simulink model "full_maneuver_platoon"  (R2022a)
settings: Solver=ode23t  StartTime=0.0  StopTime=300  FixedStep=0.1  MaxStep=0.01  RelTol=1e-3
InitFcn:
  | totalVehicles = 7;
  | if exist('vehStatesBus', 'var')==0
  | load vehBuses
  | end
  | if exist('vehErrorsBus', 'var')==0
  | load vehBuses
  | end
libraries: simulink x80, powerlib_meascontrol x16, autolibshared x7, dspsigops x4
(part 5 of 9)

== system full_maneuver_platoon/p2/CACC destination lane/Virtual Vehicle Following ==
  ego : Inport
  virtualLeader : Inport  Port=2
  leaderChange : Inport  Port=3
  extraSpaceFlag : Inport  Port=4
  Bus Selector : BusSelector  OutputSignals=u
  Compute Errors : Subsystem
  Define Desired Distance : Subsystem
  Min Velocity Control : Subsystem  TreatAsAtomicUnit=on
  NOT : Logic  Operator=NOT  IconShape=distinctive  AllPortsSameDT=off  OutDataTypeStr=boolean
  Scope : Scope  NumInputPorts=2
  Switch : Switch  Criteria=u2 > Threshold  SaturateOnIntegerOverflow=off  InputSameDT=off
  Terminator : Terminator
  Velocity Error : Subsystem
  Virtual Leader Following : Subsystem  TreatAsAtomicUnit=on
  comf saturation : Saturate  UpperLimit=maxComfAccel  LowerLimit=minComfAccel
  comf jerk : RateLimiter  RisingSlewLimit=maxComfJerk  FallingSlewLimit=minComfJerk  SampleTimeMode=inherited
  switch min vel : Subsystem
  vMin : Constant  Value=vMin
  u : Outport  InitialOutput=0  VectorParamsAs1DForOutWhenUnconnected=off
  virtualErrors : Outport  Port=2  OutputWhenDisabled=reset  InitialOutput=[0, 0]  VectorParamsAs1DForOutWhenUnconnected=off
  virtualGap : Outport  Port=3  OutputWhenDisabled=reset  InitialOutput=[0]  VectorParamsAs1DForOutWhenUnconnected=off
  wires:
  Switch/1 -> Scope/2, comf saturation/1
  comf jerk/1 -> u/1
  comf saturation/1 -> comf jerk/1
  Bus Selector/1 -> Virtual Leader Following/3(realInput)  "<u>"
  Velocity Error/2(ea) -> Min Velocity Control/2(ea)
  Velocity Error/1(ev) -> Min Velocity Control/1(ev)
  NOT/1 -> Switch/2, Scope/1, Virtual Leader Following/5(inRange)
  switch min vel/1(inRange) -> NOT/1, Min Velocity Control/3(intergralReset), Velocity Error/3(filterReset)
  extraSpaceFlag/1 -> Define Desired Distance/1(extraSpaceFlag)
  Min Velocity Control/1(u) -> Switch/3  "uMinVelControl"
  Compute Errors/3("gap ") -> virtualGap/1, switch min vel/3(gap)
  Virtual Leader Following/1(u) -> Switch/1  "uVehFoll"
  ego/1 -> Compute Errors/1(ego), Bus Selector/1, Velocity Error/1(ego)
  vMin/1 -> switch min vel/6(vRef), Velocity Error/2(velRef)
  Compute Errors/1(errors) -> switch min vel/1(errors), Virtual Leader Following/1(errors), virtualErrors/1
  virtualLeader/1 -> Compute Errors/2(leader)
  leaderChange/1 -> Compute Errors/5(velFilterReset), Virtual Leader Following/4(leaderChange)
  Compute Errors/4(unsafeFlag) -> Terminator/1
  Compute Errors/2(errorsDot) -> Virtual Leader Following/2(errorsDot), switch min vel/2(errorsDot)
  Define Desired Distance/1(h) -> switch min vel/4(h), Compute Errors/3(h)
  Define Desired Distance/2(d0) -> switch min vel/5(d0), Compute Errors/4(d0)

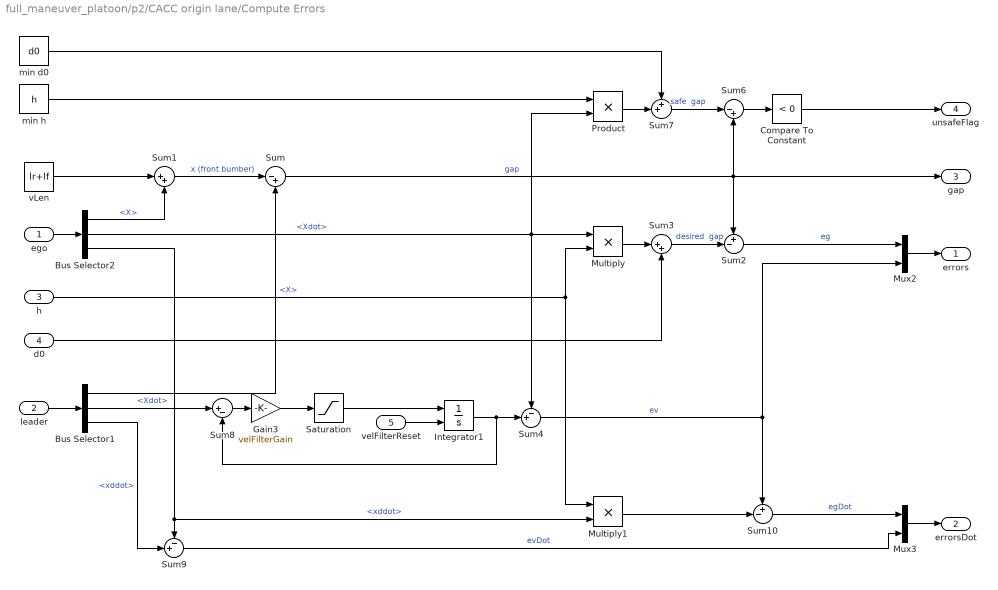
== system full_maneuver_platoon/p2/CACC origin lane/Compute Errors ==
  ego : Inport
  leader : Inport  Port=2
  h : Inport  Port=3
  d0 : Inport  Port=4
  velFilterReset : Inport  Port=5
  Bus Selector1 : BusSelector  OutputSignals=X,Xdot,xddot
  Bus Selector2 : BusSelector  OutputSignals=X,Xdot,xddot
  Compare To Constant : simulink/Logic and Bit Operations/Compare To Constant  relop=<  const=0  OutDataTypeStr=boolean
  Gain3 : Gain  Gain=velFilterGain
  Integrator1 : Integrator  ExternalReset=rising  InitialCondition=vx0
  Multiply : Product
  Multiply1 : Product
  Mux2 : Mux  Inputs=2
  Mux3 : Mux  Inputs=2
  Product : Product
  Saturation : Saturate  UpperLimit=maxAcceleration  LowerLimit=minAcceleration
  Sum : Sum  Inputs=|-+
  Sum1 : Sum  Inputs=|++
  Sum10 : Sum  Inputs=+-|
  Sum2 : Sum  Inputs=+-|
  Sum3 : Sum  Inputs=|++
  Sum4 : Sum  Inputs=-+|
  Sum6 : Sum  Inputs=|-+
  Sum7 : Sum  Inputs=++|
  Sum8 : Sum  Inputs=|+-
  Sum9 : Sum  Inputs=-+|
  min d0 : Constant  Value=d0
  min h : Constant  Value=h
  vLen : Constant  Value=lr+lf
  errors : Outport  VectorParamsAs1DForOutWhenUnconnected=off
  errorsDot : Outport  Port=2
  "gap " : Outport  Port=3  VectorParamsAs1DForOutWhenUnconnected=off
  unsafeFlag : Outport  Port=4  VectorParamsAs1DForOutWhenUnconnected=off
  wires:
  Mux2/1 -> errors/1
  velFilterReset/1 -> Integrator1/2
  Sum6/1 -> Compare To Constant/1
  Sum7/1 -> Sum6/1  "safe  gap"
  min h/1 -> Product/1
  Compare To Constant/1 -> unsafeFlag/1
  Sum2/1 -> Mux2/1  "eg"
  Bus Selector1/1 -> Sum/2  "<X>"
  Product/1 -> Sum7/2
  Sum3/1 -> Sum2/2  "desired  gap"
  Sum1/1 -> Sum/1  "x (front bumber)"
  Bus Selector2/2 -> Sum4/1, Multiply/1, Product/2  "<Xdot>"
  d0/1 -> Sum3/2
  vLen/1 -> Sum1/1
  min d0/1 -> Sum7/1
  Multiply/1 -> Sum3/1
  Sum/1 -> Sum2/1, Sum6/2, "gap "/1  "gap"
  Bus Selector2/1 -> Sum1/2  "<X>"
  h/1 -> Multiply/2, Multiply1/1
  Bus Selector1/2 -> Sum8/1  "<Xdot>"
  Sum4/1 -> Mux2/2, Sum10/1  "ev"
  Gain3/1 -> Saturation/1
  Saturation/1 -> Integrator1/1
  Integrator1/1 -> Sum4/2, Sum8/2
  Sum8/1 -> Gain3/1
  Bus Selector1/3 -> Sum9/2  "<xddot>"
  Bus Selector2/3 -> Sum9/1, Multiply1/2  "<xddot>"
  Multiply1/1 -> Sum10/2
  Sum10/1 -> Mux3/1  "egDot"
  Sum9/1 -> Mux3/2  "evDot"
  Mux3/1 -> errorsDot/1
  ego/1 -> Bus Selector2/1
  leader/1 -> Bus Selector1/1

== system full_maneuver_platoon/p2/CACC origin lane/Define Desired Distance ==
  extraSpaceFlag : Inport
  Constant : Constant  Value=h
  Constant1 : Constant  Value=d0
  Constant2 : Constant  Value=hLC
  Constant3 : Constant  Value=d0LC
  Demux : Demux  Outputs=2
  Integrator : Integrator  InitialCondition=[h d0]
  Mux : Mux  Inputs=2
  Mux1 : Mux  Inputs=2
  Saturation1 : Saturate  UpperLimit=hFilterSaturation/2  LowerLimit=-hFilterSaturation
  Sum5 : Sum  Inputs=|+-
  Switch : Switch  Criteria=u2 > Threshold  SaturateOnIntegerOverflow=off  InputSameDT=off
  hFilterGain : Gain  Gain=hFilterGain
  h : Outport
  d0 : Outport  Port=2
  wires:
  Mux/1 -> Switch/3
  Constant/1 -> Mux/1
  hFilterGain/1 -> Saturation1/1
  Constant2/1 -> Mux1/1
  Sum5/1 -> hFilterGain/1
  Mux1/1 -> Switch/1
  Switch/1 -> Sum5/1
  Constant3/1 -> Mux1/2
  Constant1/1 -> Mux/2
  extraSpaceFlag/1 -> Switch/2
  Saturation1/1 -> Integrator/1
  Integrator/1 -> Demux/1, Sum5/2
  Demux/1 -> h/1
  Demux/2 -> d0/1

== system full_maneuver_platoon/p2/CACC origin lane/Veh Following ==
  errors : Inport
  errorsDot : Inport  Port=2
  realInput : Inport  Port=3
  leaderChange : Inport  Port=4
  inRange : Inport  Port=5
  AND : Logic  IconShape=distinctive  AllPortsSameDT=off  OutDataTypeStr=boolean
  Compare To Constant : simulink/Logic and Bit Operations/Compare To Constant  relop=~=  const=0  OutDataTypeStr=boolean
  Constant : Constant  Value=Ki
  Demux : Demux  Outputs=2
  Demux1 : Demux  Outputs=2
  Gain : Gain  Gain=Ka
  Gain1 : Gain  Gain=Kdd
  Gain3 : Gain  Commented=on  Gain=10
  Integrator1 : Integrator  Commented=on  ExternalReset=either  InitialConditionSource=external  InitialCondition=vx0
  Kd : Gain  Gain=Kd
  Kp : Gain  Gain=Kp
  Saturation : Saturate  Commented=on  UpperLimit=maxComfAccel  LowerLimit=minAcceleration
  Saturation1 : Saturate  UpperLimit=maxGapError  LowerLimit=minGapError
  Scope : Scope  NumInputPorts=6
  Sum : Sum  Inputs=+-|
  Sum1 : Sum  Inputs=+++++
  Sum8 : Sum  Commented=on  Inputs=|+-
  Transport Delay : TransportDelay  DelayTime=0.1
  integralTerm : Subsystem
  u : Outport  VectorParamsAs1DForOutWhenUnconnected=off
  wires:
  AND/1 -> integralTerm/Enable
  inRange/1 -> Integrator1/2, AND/2
  Compare To Constant/1 -> AND/1
  Constant/1 -> Compare To Constant/1
  Kp/1 -> Sum1/2, Scope/2
  Gain3/1 -> Saturation/1
  Sum8/1 -> Gain3/1
  Saturation/1 -> Integrator1/1
  Integrator1/1 -> Sum8/2
  errors/1 -> Demux/1
  Saturation1/1 -> integralTerm/1(eh), Kp/1
  Demux/2 -> Kd/1  "ev"
  Kd/1 -> Sum1/3, Scope/3
  Demux/1 -> Saturation1/1  "eg"
  leaderChange/1 -> integralTerm/3(leaderChange)
  Transport Delay/1 -> Sum1/1, Scope/1
  realInput/1 -> Sum/2, Integrator1/3
  Sum/1 -> integralTerm/2(inputDiff)
  integralTerm/1(Out1) -> Transport Delay/1
  Gain1/1 -> Sum1/4, Scope/4
  Gain/1 -> Sum1/5, Scope/5
  Sum1/1 -> Sum8/1, Sum/1, Scope/6, u/1
  errorsDot/1 -> Demux1/1
  Demux1/1 -> Gain1/1  "egDot"
  Demux1/2 -> Gain/1  "evDot"

== system full_maneuver_platoon/p2/CACC origin lane/Velocity Control ==
  ev : Inport
  ea : Inport  Port=2
  integralReset : Inport  Port=3
  Abs : Abs  SaturateOnIntegerOverflow=off
  Compare To Constant : simulink/Logic and Bit Operations/Compare To Constant  relop=<  const=maxComfAccel*2  OutDataTypeStr=boolean
  Gain : Gain  Gain=velKd
  Scope : Scope  NumInputPorts=4
  Scope1 : Scope  NumInputPorts=2
  Sum3 : Sum  Inputs=+++
  Transport Delay : TransportDelay  DelayTime=0.1
  integral term : Subsystem
  velKp : Gain  Gain=velKp
  u : Outport  VectorParamsAs1DForOutWhenUnconnected=off
  wires:
  integralReset/1 -> integral term/2(integralReset)
  Sum3/1 -> Transport Delay/1, Scope/4, u/1
  Gain/1 -> Sum3/3, Scope/3  "derivative"
  ea/1 -> Gain/1
  velKp/1 -> Sum3/2, Scope/2  "proportional"
  ev/1 -> integral term/1(ev), velKp/1
  Abs/1 -> Compare To Constant/1
  integral term/1(Out1) -> Scope/1, Sum3/1  "integral"
  Compare To Constant/1 -> Scope1/2, integral term/Enable
  Transport Delay/1 -> Abs/1, Scope1/1

== system full_maneuver_platoon/p2/CACC origin lane/Velocity Error ==
  ego : Inport
  velRef : Inport  Port=2
  filterReset : Inport  Port=3
  Bus Selector : BusSelector  OutputSignals=Xdot,xddot
  Gain1 : Gain  Gain=velFilterGain
  Gain3 : Gain  Gain=velFilterGain
  Integrator1 : Integrator  ExternalReset=rising  InitialConditionSource=external  InitialCondition=vx0
  Saturation : Saturate  UpperLimit=maxComfAccel  LowerLimit=minComfAccel
  Saturation1 : Saturate  UpperLimit=maxComfAccel  LowerLimit=minComfAccel
  Scope : Scope  NumInputPorts=2
  Scope1 : Scope  NumInputPorts=2
  Sum : Sum  Inputs=+-|
  Sum1 : Sum  Inputs=-+|
  Sum2 : Sum  Inputs=+-|
  Sum8 : Sum  Inputs=|+-
  ev : Outport
  ea : Outport  Port=2
  wires:
  Saturation1/1 -> Sum2/1
  Gain1/1 -> Saturation1/1
  Sum1/1 -> Gain1/1  "filter error"
  Bus Selector/2 -> Sum2/2  "<xddot>"
  Sum2/1 -> ea/1, Scope/2
  Sum8/1 -> Gain3/1
  Gain3/1 -> Saturation/1
  Saturation/1 -> Integrator1/1
  velRef/1 -> Sum8/1, Sum1/2, Scope1/1
  Integrator1/1 -> Sum/1, Sum8/2, Sum1/1, Scope1/2
  ego/1 -> Bus Selector/1
  Bus Selector/1 -> Integrator1/3, Sum/2  "<Xdot>"
  Sum/1 -> ev/1, Scope/1
  filterReset/1 -> Integrator1/2

== system full_maneuver_platoon/p2/CACC origin lane/switch free flow ==
  errors : Inport
  errorsDot : Inport  Port=2
  gap : Inport  Port=3
  h : Inport  Port=4
  d0 : Inport  Port=5
  vRef : Inport  Port=6
  Demux1 : Demux  Outputs=2
  Gain1 : Gain
  MATLAB Function : MATLAB Function  TreatAsAtomicUnit=on
  Relay : Relay  OnSwitchValue=1  OffSwitchValue=-1
  Scope : Scope  NumInputPorts=3
  Selector : Selector  InputPortWidth=2  IndexOptions=Index vector (dialog)  Indices=[2]  OutputSizes=1
  Sum2 : Sum  Inputs=-+
  inRange : Outport  VectorParamsAs1DForOutWhenUnconnected=off
  wires:
  d0/1 -> MATLAB Function/2(d0)
  vRef/1 -> MATLAB Function/3(vRef)
  h/1 -> Gain1/1
  errors/1 -> Selector/1
  gap/1 -> Scope/1, Sum2/1
  Sum2/1 -> Relay/1
  Selector/1 -> MATLAB Function/4(ev)
  Relay/1 -> inRange/1, Scope/3
  Gain1/1 -> MATLAB Function/1(h)
  MATLAB Function/1(maxGap) -> Sum2/2, Scope/2
  errorsDot/1 -> Demux1/1
  Demux1/1 -> MATLAB Function/5(ehDot)
  Demux1/2 -> MATLAB Function/6(ea)

== system full_maneuver_platoon/p2/Find Leader/Subsystem ==
  ego : Inport
  all : Inport  Port=2
  Enable : EnablePort
  MATLAB Function : MATLAB Function  TreatAsAtomicUnit=on
  idx : Outport  InitialOutput=1  VectorParamsAs1DForOutWhenUnconnected=off
  wires:
  all/1 -> MATLAB Function/2(allVehicles)
  MATLAB Function/1(leaderIdx) -> idx/1
  ego/1 -> MATLAB Function/1(ego)

== system full_maneuver_platoon/p2/Find Leader/farAwayVeh ==
  ego : Inport  OutDataTypeStr=Bus: vehStatesBus
  Bus Assignment : BusAssignment  AssignedSignals=X
  Bus Selector : BusSelector  OutputSignals=X
  Constant : Constant  Value=1000
  Sum : Sum  Inputs=|++
  Out1 : Outport  OutDataTypeStr=Bus: vehStatesBus  VectorParamsAs1DForOutWhenUnconnected=off
  wires:
  Sum/1 -> Bus Assignment/2  "X"
  Bus Selector/1 -> Sum/1  "<X>"
  Bus Assignment/1 -> Out1/1
  Constant/1 -> Sum/2
  ego/1 -> Bus Selector/1, Bus Assignment/1

== system full_maneuver_platoon/p2/Lane Change Strategy/Strategy 1: synchronous ==
  gapRequest : Inport
  lcFlag : Inport  Port=2
  positionInPlatoon : Inport  Port=3
  platoonStates : Inport  Port=4
  isLaneChangeSafe : Inport  Port=5
  isLaneChangeDone : Inport  Port=6
  isGapClosed : Inport  Port=7
  realCACCstate : Inport  Port=8
  Chart : Stateflow chart  TreatAsAtomicUnit=on
      settings: PortSchema="{\"entries\":[{\"content\":{\"sides\":[{\"content\":{\"connectorIds\":[\"In1\",\"In2\",\"In3\",\"In4\",\"In6\",\"In5\",\"In7\",\"In8\"]},\"type\":\"ConnectorPlacement.EquallySpacedRectSide\",\"uuid\":\"395656aa-3e0f-49ff-a8a2-bf7c57c42e6d\"},{\"content\":{\"connectorIds\":[\"Out1\",\"Out2\",\"Out3\",\"Out4\",\"Out5\"],\"side\":\"RIGHT\"},\"type\":\"ConnectorPlacement.EquallySpacedRectSide\",\"uuid\":\"d914af52-9e9a-4b17-a1e4-773e769de9a6\"},{\"content\":{\"connectorIds\":[],\"side\":\"TOP\"},\"type\":\"ConnectorPlacement.EquallySpacedRectSide\",\"uuid\":\"e4221941-8de7-47a5-9bcd-f17ee6e4f42c\"}]},\"type\":\"ConnectorPlacement.EquallySpacedConnector\",\"uuid\":\"61bad5e0-e673-4247-b49d-1296c33c05b0\"}],\"packageUris\":[\"http://schema.mathworks.com/mf0/Connector/19700101\"],\"version\":\"1.0\"}"
  Sum : Sum  Inputs=|++
  Width : Width
  determine virtual follower idx : Subsystem  TreatAsAtomicUnit=on
  determine virtual leader idx : Subsystem
  number of non-lane changing vehicles : Constant  Value=4
  maneuverState : Outport
  mustIncreaseGap : Outport  Port=2
  canStartLaneChange : Outport  Port=3
  hasVirtualLeader : Outport  Port=4
  virtualLeaderIdx : Outport  Port=5
  virtualFollowerIdx : Outport  Port=6
  wires:
  Sum/1 -> determine virtual leader idx/1(nVehicles)
  Width/1 -> Sum/1
  number of non-lane changing vehicles/1 -> Sum/2
  determine virtual leader idx/1(virtualLeaderIdx) -> virtualLeaderIdx/1
  determine virtual follower idx/1(virtualFollowerIdx) -> virtualFollowerIdx/1
  isLaneChangeDone/1 -> Chart/5(isLaneChangeDone)
  positionInPlatoon/1 -> Chart/3(positionInPlatoon)
  isLaneChangeSafe/1 -> Chart/6(isLaneChangeSafe)
  lcFlag/1 -> Chart/2(hasLaneChangeIntention), determine virtual leader idx/2(lcFlag)
  Chart/2(mustIncreaseGap) -> mustIncreaseGap/1
  Chart/1(maneuverState) -> maneuverState/1
  platoonStates/1 -> Chart/4(platoonStates), Width/1
  isGapClosed/1 -> Chart/7(isGapClosed)
  Chart/3(canStartLaneChange) -> canStartLaneChange/1
  Chart/5(hasVirtualFollower) -> determine virtual follower idx/Enable
  Chart/4(hasVirtualLeader) -> determine virtual leader idx/Enable, hasVirtualLeader/1
  gapRequest/1 -> Chart/1(gapRequest)
  realCACCstate/1 -> Chart/8(realCACCstate)

== system full_maneuver_platoon/p2/Lane Change Strategy/Strategy 2: leader first ==
  gapRequest : Inport
  lcFlag : Inport  Port=2
  positionInPlatoon : Inport  Port=3
  platoonStates : Inport  Port=4
  isLaneChangeSafe : Inport  Port=5
  isLaneChangeDone : Inport  Port=6
  isGapClosed : Inport  Port=7
  realCACCstate : Inport  Port=8
  Chart : Stateflow chart  TreatAsAtomicUnit=on
      settings: PortSchema="{\"entries\":[{\"content\":{\"sides\":[{\"content\":{\"connectorIds\":[\"In1\",\"In2\",\"In3\",\"In5\",\"In4\",\"In6\",\"In7\",\"In8\"]},\"type\":\"ConnectorPlacement.EquallySpacedRectSide\",\"uuid\":\"395656aa-3e0f-49ff-a8a2-bf7c57c42e6d\"},{\"content\":{\"connectorIds\":[\"Out1\",\"Out2\",\"Out3\",\"Out4\",\"Out5\"],\"side\":\"RIGHT\"},\"type\":\"ConnectorPlacement.EquallySpacedRectSide\",\"uuid\":\"d914af52-9e9a-4b17-a1e4-773e769de9a6\"},{\"content\":{\"connectorIds\":[],\"side\":\"TOP\"},\"type\":\"ConnectorPlacement.EquallySpacedRectSide\",\"uuid\":\"e4221941-8de7-47a5-9bcd-f17ee6e4f42c\"}]},\"type\":\"ConnectorPlacement.EquallySpacedConnector\",\"uuid\":\"61bad5e0-e673-4247-b49d-1296c33c05b0\"}],\"packageUris\":[\"http://schema.mathworks.com/mf0/Connector/19700101\"],\"version\":\"1.0\"}"
  Sum : Sum  Inputs=|++
  Width : Width
  determine virtual follower idx : Subsystem  TreatAsAtomicUnit=on
  determine virtual leader idx : Subsystem
  number of non-lane changing vehicles : Constant  Value=4
  maneuverState : Outport
  mustIncreaseGap : Outport  Port=2
  canStartLaneChange : Outport  Port=3
  hasVirtualLeader : Outport  Port=4
  virtualLeaderIdx : Outport  Port=5
  virtualFollowerIdx : Outport  Port=6
  wires:
  number of non-lane changing vehicles/1 -> Sum/2
  Sum/1 -> determine virtual leader idx/1(nVehicles)
  Width/1 -> Sum/1
  determine virtual leader idx/1(virtualLeaderIdx) -> virtualLeaderIdx/1
  determine virtual follower idx/1(virtualFollowerIdx) -> virtualFollowerIdx/1
  isLaneChangeDone/1 -> Chart/5(isLaneChangeDone)
  positionInPlatoon/1 -> determine virtual leader idx/3(posInPlatoon), Chart/3(positionInPlatoon)
  isLaneChangeSafe/1 -> Chart/6(isLaneChangeSafe)
  lcFlag/1 -> determine virtual leader idx/2(lcFlag), Chart/2(hasLaneChangeIntention)
  Chart/2(mustIncreaseGap) -> mustIncreaseGap/1
  Chart/1(maneuverState) -> maneuverState/1
  platoonStates/1 -> Width/1, Chart/4(platoonStates)
  isGapClosed/1 -> Chart/7(isGapClosed)
  Chart/3(canStartLaneChange) -> canStartLaneChange/1
  Chart/5(hasVirtualFollower) -> determine virtual follower idx/Enable
  Chart/4(hasVirtualLeader) -> determine virtual leader idx/Enable, hasVirtualLeader/1
  gapRequest/1 -> Chart/1(gapRequest)
  realCACCstate/1 -> Chart/8(realCACCstate)

== system full_maneuver_platoon/p2/Lane Change Strategy/Strategy 3: last first ==
  gapRequest : Inport
  lcFlag : Inport  Port=2
  positionInPlatoon : Inport  Port=3
  platoonStates : Inport  Port=4
  isLaneChangeSafe : Inport  Port=5
  isLaneChangeDone : Inport  Port=6
  isGapClosed : Inport  Port=7
  realCACCstate : Inport  Port=8
  Chart : Stateflow chart  TreatAsAtomicUnit=on
      settings: PortSchema="{\"entries\":[{\"content\":{\"sides\":[{\"content\":{\"connectorIds\":[\"In1\",\"In2\",\"In3\",\"In4\",\"In6\",\"In5\",\"In7\",\"In8\"]},\"type\":\"ConnectorPlacement.EquallySpacedRectSide\",\"uuid\":\"395656aa-3e0f-49ff-a8a2-bf7c57c42e6d\"},{\"content\":{\"connectorIds\":[\"Out1\",\"Out2\",\"Out3\",\"Out4\",\"Out5\"],\"side\":\"RIGHT\"},\"type\":\"ConnectorPlacement.EquallySpacedRectSide\",\"uuid\":\"d914af52-9e9a-4b17-a1e4-773e769de9a6\"},{\"content\":{\"connectorIds\":[],\"side\":\"TOP\"},\"type\":\"ConnectorPlacement.EquallySpacedRectSide\",\"uuid\":\"e4221941-8de7-47a5-9bcd-f17ee6e4f42c\"}]},\"type\":\"ConnectorPlacement.EquallySpacedConnector\",\"uuid\":\"61bad5e0-e673-4247-b49d-1296c33c05b0\"}],\"packageUris\":[\"http://schema.mathworks.com/mf0/Connector/19700101\"],\"version\":\"1.0\"}"
  Sum : Sum
  Width : Width
  determine virtual follower idx : Subsystem
  determine virtual leader idx : Subsystem
  number of non-lane changing vehicles : Constant  Value=4
  maneuverState : Outport
  mustIncreaseGap : Outport  Port=2
  canStartLaneChange : Outport  Port=3
  hasVirtualLeader : Outport  Port=4
  virtualLeaderIdx : Outport  Port=5
  virtualFollowerIdx : Outport  Port=6
  wires:
  Sum/1 -> determine virtual leader idx/1(nVehicles)
  number of non-lane changing vehicles/1 -> Sum/2
  determine virtual leader idx/1(virtualLeaderIdx) -> virtualLeaderIdx/1
  determine virtual follower idx/1(virtual follower idx) -> virtualFollowerIdx/1
  Width/1 -> determine virtual follower idx/1(platoonSize), Sum/1
  isLaneChangeDone/1 -> determine virtual leader idx/3(lcDone), Chart/5(isLaneChangeDone)
  positionInPlatoon/1 -> determine virtual follower idx/2(posInPlatoon), determine virtual leader idx/4(posInPlatoon), Chart/3(positionInPlatoon)
  isLaneChangeSafe/1 -> Chart/6(isLaneChangeSafe)
  lcFlag/1 -> determine virtual leader idx/2(lcFlag), Chart/2(hasLaneChangeIntention)
  Chart/2(mustIncreaseGap) -> mustIncreaseGap/1
  Chart/1(maneuverState) -> maneuverState/1
  platoonStates/1 -> Width/1, Chart/4(platoonStates)
  isGapClosed/1 -> Chart/7(isGapClosed)
  Chart/3(canStartLaneChange) -> canStartLaneChange/1
  Chart/5(hasVirtualFollower) -> determine virtual follower idx/Enable
  Chart/4(hasVirtualLeader) -> determine virtual leader idx/Enable, hasVirtualLeader/1
  gapRequest/1 -> Chart/1(gapRequest)
  realCACCstate/1 -> Chart/8(realCACCstate)

== system full_maneuver_platoon/p2/Lane Change Strategy/Strategy 4: leader first invert ==
  gapRequest : Inport
  lcFlag : Inport  Port=2
  positionInPlatoon : Inport  Port=3
  platoonStates : Inport  Port=4
  isLaneChangeSafe : Inport  Port=5
  isLaneChangeDone : Inport  Port=6
  isGapClosed : Inport  Port=7
  realCACCstate : Inport  Port=8
  Chart : Stateflow chart  TreatAsAtomicUnit=on
      settings: PortSchema="{\"entries\":[{\"content\":{\"sides\":[{\"content\":{\"connectorIds\":[\"In1\",\"In2\",\"In3\",\"In4\",\"In6\",\"In5\",\"In7\",\"In8\"]},\"type\":\"ConnectorPlacement.EquallySpacedRectSide\",\"uuid\":\"395656aa-3e0f-49ff-a8a2-bf7c57c42e6d\"},{\"content\":{\"connectorIds\":[\"Out1\",\"Out2\",\"Out3\",\"Out4\",\"Out5\"],\"side\":\"RIGHT\"},\"type\":\"ConnectorPlacement.EquallySpacedRectSide\",\"uuid\":\"d914af52-9e9a-4b17-a1e4-773e769de9a6\"},{\"content\":{\"connectorIds\":[],\"side\":\"TOP\"},\"type\":\"ConnectorPlacement.EquallySpacedRectSide\",\"uuid\":\"e4221941-8de7-47a5-9bcd-f17ee6e4f42c\"}]},\"type\":\"ConnectorPlacement.EquallySpacedConnector\",\"uuid\":\"61bad5e0-e673-4247-b49d-1296c33c05b0\"}],\"packageUris\":[\"http://schema.mathworks.com/mf0/Connector/19700101\"],\"version\":\"1.0\"}"
  Subsystem : Subsystem
  Subsystem1 : Subsystem
  Sum : Sum  Inputs=++|
  Width : Width
  number of non-lane changing vehicles : Constant  Value=4
  maneuverState : Outport
  mustIncreaseGap : Outport  Port=2
  canStartLaneChange : Outport  Port=3
  hasVirtualLeader : Outport  Port=4
  virtualLeaderIdx : Outport  Port=5
  virtualFollowerIdx : Outport  Port=6
  wires:
  Subsystem1/1(virtualLeaderIdx) -> virtualLeaderIdx/1
  Sum/1 -> Subsystem1/1(nVehicles)
  Width/1 -> Sum/2
  number of non-lane changing vehicles/1 -> Sum/1
  Subsystem/1(virtualFollowerIdx) -> virtualFollowerIdx/1
  isLaneChangeDone/1 -> Chart/5(isLaneChangeDone), Subsystem1/3(lcDone)
  positionInPlatoon/1 -> Chart/3(positionInPlatoon), Subsystem/1(posInPlatoon), Subsystem1/4(posInPlatoon)
  isLaneChangeSafe/1 -> Chart/6(isLaneChangeSafe)
  lcFlag/1 -> Chart/2(hasLaneChangeIntention), Subsystem1/2(lcFlag)
  Chart/2(mustIncreaseGap) -> mustIncreaseGap/1
  Chart/1(maneuverState) -> maneuverState/1
  platoonStates/1 -> Chart/4(platoonStates), Width/1
  isGapClosed/1 -> Chart/7(isGapClosed)
  Chart/3(canStartLaneChange) -> canStartLaneChange/1
  Chart/5(hasVirtualFollower) -> Subsystem/Enable
  Chart/4(hasVirtualLeader) -> hasVirtualLeader/1, Subsystem1/Enable
  gapRequest/1 -> Chart/1(gapRequest)
  realCACCstate/1 -> Chart/8(realCACCstate)

== system full_maneuver_platoon/p2/Lateral Control/Full State Observer ==
  note: yhat
  note: xhat
  measuredOutputs : Inport
  delta : Inport  Port=2
  Add1 : Sum  Inputs=|-+
  Gain : Gain  Gain=B  Multiplication=Matrix(K*u)
  Gain1 : Gain  Gain=C  Multiplication=Matrix(K*u)
  Gain2 : Gain  Gain=L  Multiplication=Matrix(K*u)
  Gain3 : Gain  Gain=A  Multiplication=Matrix(K*u)
  Integrator : Integrator  InitialCondition=[y0; 0; 0; 0]
  Signal Specification : SignalSpecification  Dimensions=[size(C,1) 1]
  Sum : Sum  Inputs=+++
  xhat : Outport  VectorParamsAs1DForOutWhenUnconnected=off
  wires:
  Gain2/1 -> Sum/1
  Signal Specification/1 -> Gain2/1
  Gain3/1 -> Sum/2
  Gain/1 -> Sum/3
  delta/1 -> Gain/1
  measuredOutputs/1 -> Add1/2
  Sum/1 -> Integrator/1
  Gain1/1 -> Add1/1
  Integrator/1 -> Gain1/1, Gain3/1, xhat/1
  Add1/1 -> Signal Specification/1

== system full_maneuver_platoon/p3/CACC destination lane/Subsystem ==
  note: Filter used to smooth transition when virtual following is first activated
  u : Inport
  Gain2 : Gain  Gain=10
  Integrator : Integrator  InitialCondition=maxAcceleration+1
  Sum : Sum  Inputs=|+-
  u smooth : Outport
  wires:
  Integrator/1 -> Sum/2, u smooth/1
  Sum/1 -> Gain2/1
  u/1 -> Sum/1
  Gain2/1 -> Integrator/1

== system full_maneuver_platoon/p3/CACC destination lane/Virtual Vehicle Following ==
  ego : Inport
  virtualLeader : Inport  Port=2
  leaderChange : Inport  Port=3
  extraSpaceFlag : Inport  Port=4
  Bus Selector : BusSelector  OutputSignals=u
  Compute Errors : Subsystem
  Define Desired Distance : Subsystem
  Min Velocity Control : Subsystem  TreatAsAtomicUnit=on
  NOT : Logic  Operator=NOT  IconShape=distinctive  AllPortsSameDT=off  OutDataTypeStr=boolean
  Scope : Scope  NumInputPorts=2
  Switch : Switch  Criteria=u2 > Threshold  SaturateOnIntegerOverflow=off  InputSameDT=off
  Terminator : Terminator
  Velocity Error : Subsystem
  Virtual Leader Following : Subsystem  TreatAsAtomicUnit=on
  comf saturation : Saturate  UpperLimit=maxComfAccel  LowerLimit=minComfAccel
  comf jerk : RateLimiter  RisingSlewLimit=maxComfJerk  FallingSlewLimit=minComfJerk  SampleTimeMode=inherited
  switch min vel : Subsystem
  vMin : Constant  Value=vMin
  u : Outport  InitialOutput=0  VectorParamsAs1DForOutWhenUnconnected=off
  virtualErrors : Outport  Port=2  OutputWhenDisabled=reset  InitialOutput=[0, 0]  VectorParamsAs1DForOutWhenUnconnected=off
  virtualGap : Outport  Port=3  OutputWhenDisabled=reset  InitialOutput=[0]  VectorParamsAs1DForOutWhenUnconnected=off
  wires:
  Define Desired Distance/2(d0) -> Compute Errors/4(d0), switch min vel/5(d0)
  Define Desired Distance/1(h) -> Compute Errors/3(h), switch min vel/4(h)
  Compute Errors/2(errorsDot) -> switch min vel/2(errorsDot), Virtual Leader Following/2(errorsDot)
  Compute Errors/4(unsafeFlag) -> Terminator/1
  leaderChange/1 -> Virtual Leader Following/4(leaderChange), Compute Errors/5(velFilterReset)
  virtualLeader/1 -> Compute Errors/2(leader)
  Compute Errors/1(errors) -> virtualErrors/1, Virtual Leader Following/1(errors), switch min vel/1(errors)
  vMin/1 -> Velocity Error/2(velRef), switch min vel/6(vRef)
  ego/1 -> Velocity Error/1(ego), Bus Selector/1, Compute Errors/1(ego)
  Virtual Leader Following/1(u) -> Switch/1  "uVehFoll"
  Compute Errors/3("gap ") -> switch min vel/3(gap), virtualGap/1
  Min Velocity Control/1(u) -> Switch/3  "uMinVelControl"
  extraSpaceFlag/1 -> Define Desired Distance/1(extraSpaceFlag)
  switch min vel/1(inRange) -> Velocity Error/3(filterReset), Min Velocity Control/3(intergralReset), NOT/1
  NOT/1 -> Virtual Leader Following/5(inRange), Scope/1, Switch/2
  Velocity Error/1(ev) -> Min Velocity Control/1(ev)
  Velocity Error/2(ea) -> Min Velocity Control/2(ea)
  Bus Selector/1 -> Virtual Leader Following/3(realInput)  "<u>"
  comf saturation/1 -> comf jerk/1
  comf jerk/1 -> u/1
  Switch/1 -> comf saturation/1, Scope/2

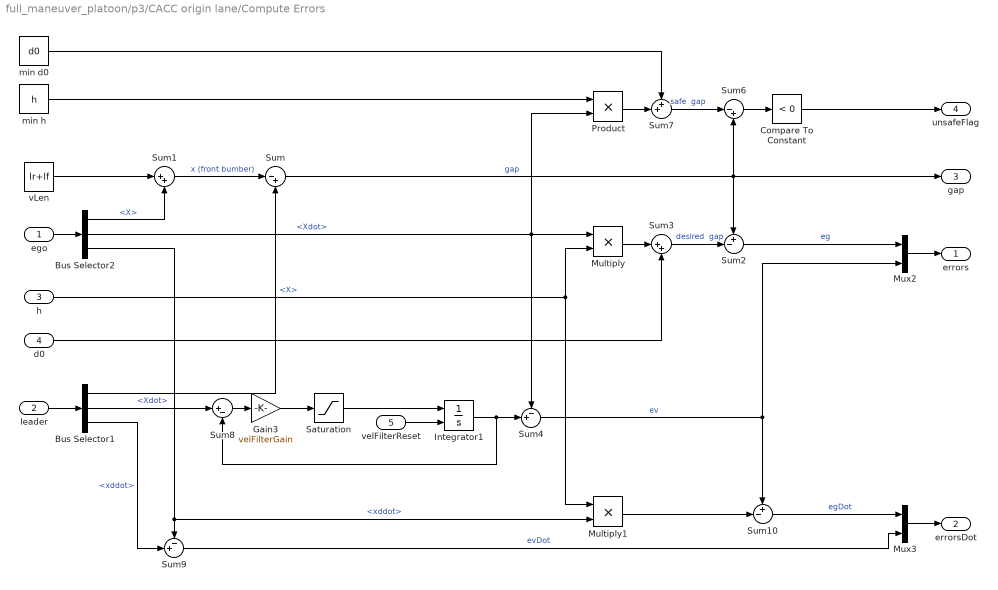
== system full_maneuver_platoon/p3/CACC origin lane/Compute Errors ==
  ego : Inport
  leader : Inport  Port=2
  h : Inport  Port=3
  d0 : Inport  Port=4
  velFilterReset : Inport  Port=5
  Bus Selector1 : BusSelector  OutputSignals=X,Xdot,xddot
  Bus Selector2 : BusSelector  OutputSignals=X,Xdot,xddot
  Compare To Constant : simulink/Logic and Bit Operations/Compare To Constant  relop=<  const=0  OutDataTypeStr=boolean
  Gain3 : Gain  Gain=velFilterGain
  Integrator1 : Integrator  ExternalReset=rising  InitialCondition=vx0
  Multiply : Product
  Multiply1 : Product
  Mux2 : Mux  Inputs=2
  Mux3 : Mux  Inputs=2
  Product : Product
  Saturation : Saturate  UpperLimit=maxAcceleration  LowerLimit=minAcceleration
  Sum : Sum  Inputs=|-+
  Sum1 : Sum  Inputs=|++
  Sum10 : Sum  Inputs=+-|
  Sum2 : Sum  Inputs=+-|
  Sum3 : Sum  Inputs=|++
  Sum4 : Sum  Inputs=-+|
  Sum6 : Sum  Inputs=|-+
  Sum7 : Sum  Inputs=++|
  Sum8 : Sum  Inputs=|+-
  Sum9 : Sum  Inputs=-+|
  min d0 : Constant  Value=d0
  min h : Constant  Value=h
  vLen : Constant  Value=lr+lf
  errors : Outport  VectorParamsAs1DForOutWhenUnconnected=off
  errorsDot : Outport  Port=2
  "gap " : Outport  Port=3  VectorParamsAs1DForOutWhenUnconnected=off
  unsafeFlag : Outport  Port=4  VectorParamsAs1DForOutWhenUnconnected=off
  wires:
  leader/1 -> Bus Selector1/1
  ego/1 -> Bus Selector2/1
  Mux3/1 -> errorsDot/1
  Sum9/1 -> Mux3/2  "evDot"
  Sum10/1 -> Mux3/1  "egDot"
  Multiply1/1 -> Sum10/2
  Bus Selector2/3 -> Multiply1/2, Sum9/1  "<xddot>"
  Bus Selector1/3 -> Sum9/2  "<xddot>"
  Sum8/1 -> Gain3/1
  Integrator1/1 -> Sum8/2, Sum4/2
  Saturation/1 -> Integrator1/1
  Gain3/1 -> Saturation/1
  Sum4/1 -> Sum10/1, Mux2/2  "ev"
  Bus Selector1/2 -> Sum8/1  "<Xdot>"
  h/1 -> Multiply1/1, Multiply/2
  Bus Selector2/1 -> Sum1/2  "<X>"
  Sum/1 -> "gap "/1, Sum6/2, Sum2/1  "gap"
  Multiply/1 -> Sum3/1
  min d0/1 -> Sum7/1
  vLen/1 -> Sum1/1
  d0/1 -> Sum3/2
  Bus Selector2/2 -> Product/2, Multiply/1, Sum4/1  "<Xdot>"
  Sum1/1 -> Sum/1  "x (front bumber)"
  Sum3/1 -> Sum2/2  "desired  gap"
  Product/1 -> Sum7/2
  Bus Selector1/1 -> Sum/2  "<X>"
  Sum2/1 -> Mux2/1  "eg"
  Compare To Constant/1 -> unsafeFlag/1
  min h/1 -> Product/1
  Sum7/1 -> Sum6/1  "safe  gap"
  Sum6/1 -> Compare To Constant/1
  velFilterReset/1 -> Integrator1/2
  Mux2/1 -> errors/1

== system full_maneuver_platoon/p3/CACC origin lane/Define Desired Distance ==
  extraSpaceFlag : Inport
  Constant : Constant  Value=h
  Constant1 : Constant  Value=d0
  Constant2 : Constant  Value=hLC
  Constant3 : Constant  Value=d0LC
  Demux : Demux  Outputs=2
  Integrator : Integrator  InitialCondition=[h d0]
  Mux : Mux  Inputs=2
  Mux1 : Mux  Inputs=2
  Saturation1 : Saturate  UpperLimit=hFilterSaturation/2  LowerLimit=-hFilterSaturation
  Sum5 : Sum  Inputs=|+-
  Switch : Switch  Criteria=u2 > Threshold  SaturateOnIntegerOverflow=off  InputSameDT=off
  hFilterGain : Gain  Gain=hFilterGain
  h : Outport
  d0 : Outport  Port=2
  wires:
  Demux/2 -> d0/1
  Demux/1 -> h/1
  Integrator/1 -> Sum5/2, Demux/1
  Saturation1/1 -> Integrator/1
  extraSpaceFlag/1 -> Switch/2
  Constant1/1 -> Mux/2
  Constant3/1 -> Mux1/2
  Switch/1 -> Sum5/1
  Mux1/1 -> Switch/1
  Sum5/1 -> hFilterGain/1
  Constant2/1 -> Mux1/1
  hFilterGain/1 -> Saturation1/1
  Constant/1 -> Mux/1
  Mux/1 -> Switch/3

== system full_maneuver_platoon/p3/CACC origin lane/Veh Following ==
  errors : Inport
  errorsDot : Inport  Port=2
  realInput : Inport  Port=3
  leaderChange : Inport  Port=4
  inRange : Inport  Port=5
  AND : Logic  IconShape=distinctive  AllPortsSameDT=off  OutDataTypeStr=boolean
  Compare To Constant : simulink/Logic and Bit Operations/Compare To Constant  relop=~=  const=0  OutDataTypeStr=boolean
  Constant : Constant  Value=Ki
  Demux : Demux  Outputs=2
  Demux1 : Demux  Outputs=2
  Gain : Gain  Gain=Ka
  Gain1 : Gain  Gain=Kdd
  Gain3 : Gain  Commented=on  Gain=10
  Integrator1 : Integrator  Commented=on  ExternalReset=either  InitialConditionSource=external  InitialCondition=vx0
  Kd : Gain  Gain=Kd
  Kp : Gain  Gain=Kp
  Saturation : Saturate  Commented=on  UpperLimit=maxComfAccel  LowerLimit=minAcceleration
  Saturation1 : Saturate  UpperLimit=maxGapError  LowerLimit=minGapError
  Scope : Scope  NumInputPorts=6
  Sum : Sum  Inputs=+-|
  Sum1 : Sum  Inputs=+++++
  Sum8 : Sum  Commented=on  Inputs=|+-
  Transport Delay : TransportDelay  DelayTime=0.1
  integralTerm : Subsystem
  u : Outport  VectorParamsAs1DForOutWhenUnconnected=off
  wires:
  Demux1/2 -> Gain/1  "evDot"
  Demux1/1 -> Gain1/1  "egDot"
  errorsDot/1 -> Demux1/1
  Sum1/1 -> u/1, Scope/6, Sum/1, Sum8/1
  Gain/1 -> Scope/5, Sum1/5
  Gain1/1 -> Scope/4, Sum1/4
  integralTerm/1(Out1) -> Transport Delay/1
  Sum/1 -> integralTerm/2(inputDiff)
  realInput/1 -> Integrator1/3, Sum/2
  Transport Delay/1 -> Scope/1, Sum1/1
  leaderChange/1 -> integralTerm/3(leaderChange)
  Demux/1 -> Saturation1/1  "eg"
  Kd/1 -> Scope/3, Sum1/3
  Demux/2 -> Kd/1  "ev"
  Saturation1/1 -> Kp/1, integralTerm/1(eh)
  errors/1 -> Demux/1
  Integrator1/1 -> Sum8/2
  Saturation/1 -> Integrator1/1
  Sum8/1 -> Gain3/1
  Gain3/1 -> Saturation/1
  Kp/1 -> Scope/2, Sum1/2
  Constant/1 -> Compare To Constant/1
  Compare To Constant/1 -> AND/1
  inRange/1 -> AND/2, Integrator1/2
  AND/1 -> integralTerm/Enable

== system full_maneuver_platoon/p3/CACC origin lane/Velocity Control ==
  ev : Inport
  ea : Inport  Port=2
  integralReset : Inport  Port=3
  Abs : Abs  SaturateOnIntegerOverflow=off
  Compare To Constant : simulink/Logic and Bit Operations/Compare To Constant  relop=<  const=maxComfAccel*2  OutDataTypeStr=boolean
  Gain : Gain  Gain=velKd
  Scope : Scope  NumInputPorts=4
  Scope1 : Scope  NumInputPorts=2
  Sum3 : Sum  Inputs=+++
  Transport Delay : TransportDelay  DelayTime=0.1
  integral term : Subsystem
  velKp : Gain  Gain=velKp
  u : Outport  VectorParamsAs1DForOutWhenUnconnected=off
  wires:
  Transport Delay/1 -> Scope1/1, Abs/1
  Compare To Constant/1 -> integral term/Enable, Scope1/2
  integral term/1(Out1) -> Sum3/1, Scope/1  "integral"
  Abs/1 -> Compare To Constant/1
  ev/1 -> velKp/1, integral term/1(ev)
  velKp/1 -> Scope/2, Sum3/2  "proportional"
  ea/1 -> Gain/1
  Gain/1 -> Scope/3, Sum3/3  "derivative"
  Sum3/1 -> u/1, Scope/4, Transport Delay/1
  integralReset/1 -> integral term/2(integralReset)

== system full_maneuver_platoon/p3/CACC origin lane/Velocity Error ==
  ego : Inport
  velRef : Inport  Port=2
  filterReset : Inport  Port=3
  Bus Selector : BusSelector  OutputSignals=Xdot,xddot
  Gain1 : Gain  Gain=velFilterGain
  Gain3 : Gain  Gain=velFilterGain
  Integrator1 : Integrator  ExternalReset=rising  InitialConditionSource=external  InitialCondition=vx0
  Saturation : Saturate  UpperLimit=maxComfAccel  LowerLimit=minComfAccel
  Saturation1 : Saturate  UpperLimit=maxComfAccel  LowerLimit=minComfAccel
  Scope : Scope  NumInputPorts=2
  Scope1 : Scope  NumInputPorts=2
  Sum : Sum  Inputs=+-|
  Sum1 : Sum  Inputs=-+|
  Sum2 : Sum  Inputs=+-|
  Sum8 : Sum  Inputs=|+-
  ev : Outport
  ea : Outport  Port=2
  wires:
  filterReset/1 -> Integrator1/2
  Sum/1 -> Scope/1, ev/1
  Bus Selector/1 -> Sum/2, Integrator1/3  "<Xdot>"
  ego/1 -> Bus Selector/1
  Integrator1/1 -> Scope1/2, Sum1/1, Sum8/2, Sum/1
  velRef/1 -> Scope1/1, Sum1/2, Sum8/1
  Saturation/1 -> Integrator1/1
  Gain3/1 -> Saturation/1
  Sum8/1 -> Gain3/1
  Sum2/1 -> Scope/2, ea/1
  Bus Selector/2 -> Sum2/2  "<xddot>"
  Sum1/1 -> Gain1/1  "filter error"
  Gain1/1 -> Saturation1/1
  Saturation1/1 -> Sum2/1

== system full_maneuver_platoon/p3/CACC origin lane/switch free flow ==
  errors : Inport
  errorsDot : Inport  Port=2
  gap : Inport  Port=3
  h : Inport  Port=4
  d0 : Inport  Port=5
  vRef : Inport  Port=6
  Demux1 : Demux  Outputs=2
  Gain1 : Gain
  MATLAB Function : MATLAB Function  TreatAsAtomicUnit=on
  Relay : Relay  OnSwitchValue=1  OffSwitchValue=-1
  Scope : Scope  NumInputPorts=3
  Selector : Selector  InputPortWidth=2  IndexOptions=Index vector (dialog)  Indices=[2]  OutputSizes=1
  Sum2 : Sum  Inputs=-+
  inRange : Outport  VectorParamsAs1DForOutWhenUnconnected=off
  wires:
  Demux1/2 -> MATLAB Function/6(ea)
  Demux1/1 -> MATLAB Function/5(ehDot)
  errorsDot/1 -> Demux1/1
  MATLAB Function/1(maxGap) -> Scope/2, Sum2/2
  Gain1/1 -> MATLAB Function/1(h)
  Relay/1 -> Scope/3, inRange/1
  Selector/1 -> MATLAB Function/4(ev)
  Sum2/1 -> Relay/1
  gap/1 -> Sum2/1, Scope/1
  errors/1 -> Selector/1
  h/1 -> Gain1/1
  vRef/1 -> MATLAB Function/3(vRef)
  d0/1 -> MATLAB Function/2(d0)

== system full_maneuver_platoon/p3/Find Leader/Subsystem ==
  ego : Inport
  all : Inport  Port=2
  Enable : EnablePort
  MATLAB Function : MATLAB Function  TreatAsAtomicUnit=on
  idx : Outport  InitialOutput=1  VectorParamsAs1DForOutWhenUnconnected=off
  wires:
  ego/1 -> MATLAB Function/1(ego)
  MATLAB Function/1(leaderIdx) -> idx/1
  all/1 -> MATLAB Function/2(allVehicles)

== system full_maneuver_platoon/p3/Find Leader/farAwayVeh ==
  ego : Inport  OutDataTypeStr=Bus: vehStatesBus
  Bus Assignment : BusAssignment  AssignedSignals=X
  Bus Selector : BusSelector  OutputSignals=X
  Constant : Constant  Value=1000
  Sum : Sum  Inputs=|++
  Out1 : Outport  OutDataTypeStr=Bus: vehStatesBus  VectorParamsAs1DForOutWhenUnconnected=off
  wires:
  ego/1 -> Bus Assignment/1, Bus Selector/1
  Constant/1 -> Sum/2
  Bus Assignment/1 -> Out1/1
  Bus Selector/1 -> Sum/1  "<X>"
  Sum/1 -> Bus Assignment/2  "X"

== system full_maneuver_platoon/p3/Lane Change Strategy/Strategy 1: synchronous ==
  gapRequest : Inport
  lcFlag : Inport  Port=2
  positionInPlatoon : Inport  Port=3
  platoonStates : Inport  Port=4
  isLaneChangeSafe : Inport  Port=5
  isLaneChangeDone : Inport  Port=6
  isGapClosed : Inport  Port=7
  realCACCstate : Inport  Port=8
  Chart : Stateflow chart  TreatAsAtomicUnit=on
      settings: PortSchema="{\"entries\":[{\"content\":{\"sides\":[{\"content\":{\"connectorIds\":[\"In1\",\"In2\",\"In3\",\"In4\",\"In6\",\"In5\",\"In7\",\"In8\"]},\"type\":\"ConnectorPlacement.EquallySpacedRectSide\",\"uuid\":\"395656aa-3e0f-49ff-a8a2-bf7c57c42e6d\"},{\"content\":{\"connectorIds\":[\"Out1\",\"Out2\",\"Out3\",\"Out4\",\"Out5\"],\"side\":\"RIGHT\"},\"type\":\"ConnectorPlacement.EquallySpacedRectSide\",\"uuid\":\"d914af52-9e9a-4b17-a1e4-773e769de9a6\"},{\"content\":{\"connectorIds\":[],\"side\":\"TOP\"},\"type\":\"ConnectorPlacement.EquallySpacedRectSide\",\"uuid\":\"e4221941-8de7-47a5-9bcd-f17ee6e4f42c\"}]},\"type\":\"ConnectorPlacement.EquallySpacedConnector\",\"uuid\":\"61bad5e0-e673-4247-b49d-1296c33c05b0\"}],\"packageUris\":[\"http://schema.mathworks.com/mf0/Connector/19700101\"],\"version\":\"1.0\"}"
  Sum : Sum  Inputs=|++
  Width : Width
  determine virtual follower idx : Subsystem  TreatAsAtomicUnit=on
  determine virtual leader idx : Subsystem
  number of non-lane changing vehicles : Constant  Value=4
  maneuverState : Outport
  mustIncreaseGap : Outport  Port=2
  canStartLaneChange : Outport  Port=3
  hasVirtualLeader : Outport  Port=4
  virtualLeaderIdx : Outport  Port=5
  virtualFollowerIdx : Outport  Port=6
  wires:
  realCACCstate/1 -> Chart/8(realCACCstate)
  gapRequest/1 -> Chart/1(gapRequest)
  Chart/4(hasVirtualLeader) -> hasVirtualLeader/1, determine virtual leader idx/Enable
  Chart/5(hasVirtualFollower) -> determine virtual follower idx/Enable
  Chart/3(canStartLaneChange) -> canStartLaneChange/1
  isGapClosed/1 -> Chart/7(isGapClosed)
  platoonStates/1 -> Width/1, Chart/4(platoonStates)
  Chart/1(maneuverState) -> maneuverState/1
  Chart/2(mustIncreaseGap) -> mustIncreaseGap/1
  lcFlag/1 -> determine virtual leader idx/2(lcFlag), Chart/2(hasLaneChangeIntention)
  isLaneChangeSafe/1 -> Chart/6(isLaneChangeSafe)
  positionInPlatoon/1 -> Chart/3(positionInPlatoon)
  isLaneChangeDone/1 -> Chart/5(isLaneChangeDone)
  determine virtual follower idx/1(virtualFollowerIdx) -> virtualFollowerIdx/1
  determine virtual leader idx/1(virtualLeaderIdx) -> virtualLeaderIdx/1
  number of non-lane changing vehicles/1 -> Sum/2
  Width/1 -> Sum/1
  Sum/1 -> determine virtual leader idx/1(nVehicles)

== system full_maneuver_platoon/p3/Lane Change Strategy/Strategy 2: leader first ==
  gapRequest : Inport
  lcFlag : Inport  Port=2
  positionInPlatoon : Inport  Port=3
  platoonStates : Inport  Port=4
  isLaneChangeSafe : Inport  Port=5
  isLaneChangeDone : Inport  Port=6
  isGapClosed : Inport  Port=7
  realCACCstate : Inport  Port=8
  Chart : Stateflow chart  TreatAsAtomicUnit=on
      settings: PortSchema="{\"entries\":[{\"content\":{\"sides\":[{\"content\":{\"connectorIds\":[\"In1\",\"In2\",\"In3\",\"In5\",\"In4\",\"In6\",\"In7\",\"In8\"]},\"type\":\"ConnectorPlacement.EquallySpacedRectSide\",\"uuid\":\"395656aa-3e0f-49ff-a8a2-bf7c57c42e6d\"},{\"content\":{\"connectorIds\":[\"Out1\",\"Out2\",\"Out3\",\"Out4\",\"Out5\"],\"side\":\"RIGHT\"},\"type\":\"ConnectorPlacement.EquallySpacedRectSide\",\"uuid\":\"d914af52-9e9a-4b17-a1e4-773e769de9a6\"},{\"content\":{\"connectorIds\":[],\"side\":\"TOP\"},\"type\":\"ConnectorPlacement.EquallySpacedRectSide\",\"uuid\":\"e4221941-8de7-47a5-9bcd-f17ee6e4f42c\"}]},\"type\":\"ConnectorPlacement.EquallySpacedConnector\",\"uuid\":\"61bad5e0-e673-4247-b49d-1296c33c05b0\"}],\"packageUris\":[\"http://schema.mathworks.com/mf0/Connector/19700101\"],\"version\":\"1.0\"}"
  Sum : Sum  Inputs=|++
  Width : Width
  determine virtual follower idx : Subsystem  TreatAsAtomicUnit=on
  determine virtual leader idx : Subsystem
  number of non-lane changing vehicles : Constant  Value=4
  maneuverState : Outport
  mustIncreaseGap : Outport  Port=2
  canStartLaneChange : Outport  Port=3
  hasVirtualLeader : Outport  Port=4
  virtualLeaderIdx : Outport  Port=5
  virtualFollowerIdx : Outport  Port=6
  wires:
  realCACCstate/1 -> Chart/8(realCACCstate)
  gapRequest/1 -> Chart/1(gapRequest)
  Chart/4(hasVirtualLeader) -> hasVirtualLeader/1, determine virtual leader idx/Enable
  Chart/5(hasVirtualFollower) -> determine virtual follower idx/Enable
  Chart/3(canStartLaneChange) -> canStartLaneChange/1
  isGapClosed/1 -> Chart/7(isGapClosed)
  platoonStates/1 -> Chart/4(platoonStates), Width/1
  Chart/1(maneuverState) -> maneuverState/1
  Chart/2(mustIncreaseGap) -> mustIncreaseGap/1
  lcFlag/1 -> Chart/2(hasLaneChangeIntention), determine virtual leader idx/2(lcFlag)
  isLaneChangeSafe/1 -> Chart/6(isLaneChangeSafe)
  positionInPlatoon/1 -> Chart/3(positionInPlatoon), determine virtual leader idx/3(posInPlatoon)
  isLaneChangeDone/1 -> Chart/5(isLaneChangeDone)
  determine virtual follower idx/1(virtualFollowerIdx) -> virtualFollowerIdx/1
  determine virtual leader idx/1(virtualLeaderIdx) -> virtualLeaderIdx/1
  Width/1 -> Sum/1
  Sum/1 -> determine virtual leader idx/1(nVehicles)
  number of non-lane changing vehicles/1 -> Sum/2

== system full_maneuver_platoon/p3/Lane Change Strategy/Strategy 3: last first ==
  gapRequest : Inport
  lcFlag : Inport  Port=2
  positionInPlatoon : Inport  Port=3
  platoonStates : Inport  Port=4
  isLaneChangeSafe : Inport  Port=5
  isLaneChangeDone : Inport  Port=6
  isGapClosed : Inport  Port=7
  realCACCstate : Inport  Port=8
  Chart : Stateflow chart  TreatAsAtomicUnit=on
      settings: PortSchema="{\"entries\":[{\"content\":{\"sides\":[{\"content\":{\"connectorIds\":[\"In1\",\"In2\",\"In3\",\"In4\",\"In6\",\"In5\",\"In7\",\"In8\"]},\"type\":\"ConnectorPlacement.EquallySpacedRectSide\",\"uuid\":\"395656aa-3e0f-49ff-a8a2-bf7c57c42e6d\"},{\"content\":{\"connectorIds\":[\"Out1\",\"Out2\",\"Out3\",\"Out4\",\"Out5\"],\"side\":\"RIGHT\"},\"type\":\"ConnectorPlacement.EquallySpacedRectSide\",\"uuid\":\"d914af52-9e9a-4b17-a1e4-773e769de9a6\"},{\"content\":{\"connectorIds\":[],\"side\":\"TOP\"},\"type\":\"ConnectorPlacement.EquallySpacedRectSide\",\"uuid\":\"e4221941-8de7-47a5-9bcd-f17ee6e4f42c\"}]},\"type\":\"ConnectorPlacement.EquallySpacedConnector\",\"uuid\":\"61bad5e0-e673-4247-b49d-1296c33c05b0\"}],\"packageUris\":[\"http://schema.mathworks.com/mf0/Connector/19700101\"],\"version\":\"1.0\"}"
  Sum : Sum
  Width : Width
  determine virtual follower idx : Subsystem
  determine virtual leader idx : Subsystem
  number of non-lane changing vehicles : Constant  Value=4
  maneuverState : Outport
  mustIncreaseGap : Outport  Port=2
  canStartLaneChange : Outport  Port=3
  hasVirtualLeader : Outport  Port=4
  virtualLeaderIdx : Outport  Port=5
  virtualFollowerIdx : Outport  Port=6
  wires:
  realCACCstate/1 -> Chart/8(realCACCstate)
  gapRequest/1 -> Chart/1(gapRequest)
  Chart/4(hasVirtualLeader) -> hasVirtualLeader/1, determine virtual leader idx/Enable
  Chart/5(hasVirtualFollower) -> determine virtual follower idx/Enable
  Chart/3(canStartLaneChange) -> canStartLaneChange/1
  isGapClosed/1 -> Chart/7(isGapClosed)
  platoonStates/1 -> Chart/4(platoonStates), Width/1
  Chart/1(maneuverState) -> maneuverState/1
  Chart/2(mustIncreaseGap) -> mustIncreaseGap/1
  lcFlag/1 -> Chart/2(hasLaneChangeIntention), determine virtual leader idx/2(lcFlag)
  isLaneChangeSafe/1 -> Chart/6(isLaneChangeSafe)
  positionInPlatoon/1 -> Chart/3(positionInPlatoon), determine virtual leader idx/4(posInPlatoon), determine virtual follower idx/2(posInPlatoon)
  isLaneChangeDone/1 -> Chart/5(isLaneChangeDone), determine virtual leader idx/3(lcDone)
  Width/1 -> Sum/1, determine virtual follower idx/1(platoonSize)
  determine virtual follower idx/1(virtual follower idx) -> virtualFollowerIdx/1
  determine virtual leader idx/1(virtualLeaderIdx) -> virtualLeaderIdx/1
  number of non-lane changing vehicles/1 -> Sum/2
  Sum/1 -> determine virtual leader idx/1(nVehicles)

== system full_maneuver_platoon/p3/Lane Change Strategy/Strategy 4: leader first invert ==
  gapRequest : Inport
  lcFlag : Inport  Port=2
  positionInPlatoon : Inport  Port=3
  platoonStates : Inport  Port=4
  isLaneChangeSafe : Inport  Port=5
  isLaneChangeDone : Inport  Port=6
  isGapClosed : Inport  Port=7
  realCACCstate : Inport  Port=8
  Chart : Stateflow chart  TreatAsAtomicUnit=on
      settings: PortSchema="{\"entries\":[{\"content\":{\"sides\":[{\"content\":{\"connectorIds\":[\"In1\",\"In2\",\"In3\",\"In4\",\"In6\",\"In5\",\"In7\",\"In8\"]},\"type\":\"ConnectorPlacement.EquallySpacedRectSide\",\"uuid\":\"395656aa-3e0f-49ff-a8a2-bf7c57c42e6d\"},{\"content\":{\"connectorIds\":[\"Out1\",\"Out2\",\"Out3\",\"Out4\",\"Out5\"],\"side\":\"RIGHT\"},\"type\":\"ConnectorPlacement.EquallySpacedRectSide\",\"uuid\":\"d914af52-9e9a-4b17-a1e4-773e769de9a6\"},{\"content\":{\"connectorIds\":[],\"side\":\"TOP\"},\"type\":\"ConnectorPlacement.EquallySpacedRectSide\",\"uuid\":\"e4221941-8de7-47a5-9bcd-f17ee6e4f42c\"}]},\"type\":\"ConnectorPlacement.EquallySpacedConnector\",\"uuid\":\"61bad5e0-e673-4247-b49d-1296c33c05b0\"}],\"packageUris\":[\"http://schema.mathworks.com/mf0/Connector/19700101\"],\"version\":\"1.0\"}"
  Subsystem : Subsystem
  Subsystem1 : Subsystem
  Sum : Sum  Inputs=++|
  Width : Width
  number of non-lane changing vehicles : Constant  Value=4
  maneuverState : Outport
  mustIncreaseGap : Outport  Port=2
  canStartLaneChange : Outport  Port=3
  hasVirtualLeader : Outport  Port=4
  virtualLeaderIdx : Outport  Port=5
  virtualFollowerIdx : Outport  Port=6
  wires:
  realCACCstate/1 -> Chart/8(realCACCstate)
  gapRequest/1 -> Chart/1(gapRequest)
  Chart/4(hasVirtualLeader) -> Subsystem1/Enable, hasVirtualLeader/1
  Chart/5(hasVirtualFollower) -> Subsystem/Enable
  Chart/3(canStartLaneChange) -> canStartLaneChange/1
  isGapClosed/1 -> Chart/7(isGapClosed)
  platoonStates/1 -> Width/1, Chart/4(platoonStates)
  Chart/1(maneuverState) -> maneuverState/1
  Chart/2(mustIncreaseGap) -> mustIncreaseGap/1
  lcFlag/1 -> Subsystem1/2(lcFlag), Chart/2(hasLaneChangeIntention)
  isLaneChangeSafe/1 -> Chart/6(isLaneChangeSafe)
  positionInPlatoon/1 -> Subsystem1/4(posInPlatoon), Subsystem/1(posInPlatoon), Chart/3(positionInPlatoon)
  isLaneChangeDone/1 -> Subsystem1/3(lcDone), Chart/5(isLaneChangeDone)
  Subsystem/1(virtualFollowerIdx) -> virtualFollowerIdx/1
  number of non-lane changing vehicles/1 -> Sum/1
  Width/1 -> Sum/2
  Sum/1 -> Subsystem1/1(nVehicles)
  Subsystem1/1(virtualLeaderIdx) -> virtualLeaderIdx/1

== system full_maneuver_platoon/p3/Lateral Control/Full State Observer ==
  note: xhat
  note: yhat
  measuredOutputs : Inport
  delta : Inport  Port=2
  Add1 : Sum  Inputs=|-+
  Gain : Gain  Gain=B  Multiplication=Matrix(K*u)
  Gain1 : Gain  Gain=C  Multiplication=Matrix(K*u)
  Gain2 : Gain  Gain=L  Multiplication=Matrix(K*u)
  Gain3 : Gain  Gain=A  Multiplication=Matrix(K*u)
  Integrator : Integrator  InitialCondition=[y0; 0; 0; 0]
  Signal Specification : SignalSpecification  Dimensions=[size(C,1) 1]
  Sum : Sum  Inputs=+++
  xhat : Outport  VectorParamsAs1DForOutWhenUnconnected=off
  wires:
  Add1/1 -> Signal Specification/1
  Integrator/1 -> xhat/1, Gain3/1, Gain1/1
  Gain1/1 -> Add1/1
  Sum/1 -> Integrator/1
  measuredOutputs/1 -> Add1/2
  delta/1 -> Gain/1
  Gain/1 -> Sum/3
  Gain3/1 -> Sum/2
  Signal Specification/1 -> Gain2/1
  Gain2/1 -> Sum/1
